simulink model "bh_control_design_sandpit"  (R2016b)
settings: Solver=ode4  StartTime=0.0  StopTime=3  FixedStep=0.001  RelTol=1e-5
libraries: simulink_extras x20, simulink x10, cstblocks x5
settings Model: Creator=bhorton  LastModifiedBy=bhorton
settings SolverCC: ZeroCrossAlgorithm=Adaptive
settings OptimizationCC: LifeSpan=inf
settings DebuggingCC: SFUnexpectedBacktrackingDiag=warning  SFNoUnconditionalDefaultTransitionDiag=warning  SFExecutionAtInitializationDiag=none
settings GRTTargetCC: TargetLangStandard=C89/C90 (ANSI)
settings ConfigComp: CovMetricSettings=dw  CovHtmlReporting=on  CovSaveCumulativeToWorkspaceVar=on  CovSaveSingleToWorkspaceVar=on  CovExternalEMLEnable=off
settings SimscapeCC: SimscapeLogType=all  SimscapeLogDataHistory=10000  SelectedTab=Simscape Multibody
settings ExplorerConfigSet: InternalSimMechanicsExplorerSettings="<ExplorerConfiguration><canonicalview>default</canonicalview><AnimationSetting><BasePlaybackSpeed>1.0</BasePlaybackSpeed><PlaybackSpeedFactor>1.0</PlaybackSpeedFactor></AnimationSetting><TilePanel><TileInfo><Tiles Columns=\"2\" Count=\"4\" Rows=\"2\"><Column Left=\"2\" Weight=\"0.4992\"/><Column Left=\"655\" Weight=\"0.5008\"/><Column Left=\"1310\"/><Row Top=\"2\" Weight=\"0.4984\"/><Row Top=\"475\" Weight=\"0.5016\"/><Row Top=\"950\"/><Tile Height=\"1\" Width=\"1\" X=\"0\" Y=\"0\"/><Tile Height=\"1\" Width=\"1\" X=\"0\" Y=\"1\"/><Tile Height=\"1\" Width=\"1\" X=\"1\" Y=\"0\"/><Tile Height=\"1\" Width=\"1\" X=\"1\" Y=\"1\"/></Tiles></TileInfo><SceneInfo><SceneViewer><BGColor><R>0.60000002384185791</R><G>0.60000002384185791</G><B>0.60000002384185791</B></BGColor><Camera><DoPerspective>off</DoPerspective><Position><X>0.57010570867346566</X><Y>-0.81939487187068383</Y><Z>-0.041325690013103822</Z></Position><Center><X>0.57010570867346566</X><Y>0.37243777720020188</Y><Z>-0.041325690013103822</Z></Center><Up><X>0</X><Y>-0</Y><Z>1</Z></Up><ViewLimDist>1</ViewLimDist><YLim>0.58387397231837834</YLim><XLim>0.8103768064074045</XLim></Camera></SceneViewer><SceneViewer><BGColor><R>0.60000002384185791</R><G>0.60000002384185791</G><B>0.60000002384185791</B></BGColor><Camera><DoPerspective>off</DoPerspective><Position><X>0.51388092361444482</X><Y>0.52196280048326149</Y><Z>0.82022286793681332</Z></Position><Center><X>0.51388092361444482</X><Y>0.52196280048326149</Y><Z>-0.17977713206318668</Z></Center><Up><X>0</X><Y>1</Y><Z>-0</Z></Up><ViewLimDist>1</ViewLimDist><YLim>0.97737746692739225</YLim><XLim>1.3507104907751943</XLim></Camera></SceneViewer><SceneViewer><BGColor><R>0.60000002384185791</R><G>0.60000002384185791</G><B>0.60000002384185791</B></BGColor><Camera><DoPerspective>off</DoPerspective><Position><X>1.5094114010486579</X><Y>0.67796186035410533</Y><Z>-0.0082694811079057073</Z></Position><Center><X>0.47943838776152692</X><Y>0.67796186035410533</Y><Z>-0.0082694811079057073</Z></Center><Up><X>-0</X><Y>0</Y><Z>1</Z></Up><ViewLimDist>1</ViewLimDist><YLim>0.68608550995197048</YLim><XLim>0.95519663670037269</XLim></Camera></SceneViewer><SceneViewer><BGColor><R>0.60000002384185791</R><G>0.60000002384185791</G><B>0.60000002384185791</B></BGColor><Camera><DoPerspective>off</DoPerspective><Position><X>1.2860411296222924</X><Y>0.12259966358168611</Y><Z>0.94383913066063729</Z></Position><Center><X>0.57516484098717713</X><Y>0.83347595221680226</Y><Z>0.23296284202552392</Z></Center><Up><X>-0.40824829046386307</X><Y>0.40824829046386307</Y><Z>0.81649658092772615</Z></Up><ViewLimDist>1</ViewLimDist><YLim>0.94664886749230226</YLim><XLim>1.3123072283262387</XLim></Camera></SceneViewer></SceneInfo></TilePanel><MechEditorPanel><Cameras/><GfxPanelCameraMap/><VideoCreator><PlaybackSpeedRatio>1.0</PlaybackSpeedRatio><FrameRate>30</FrameRate><VideoFormat>Motion JPEG AVI</VideoFormat><FrameSize>auto</FrameSize></VideoCreator></MechEditorPanel></ExplorerConfiguration>"

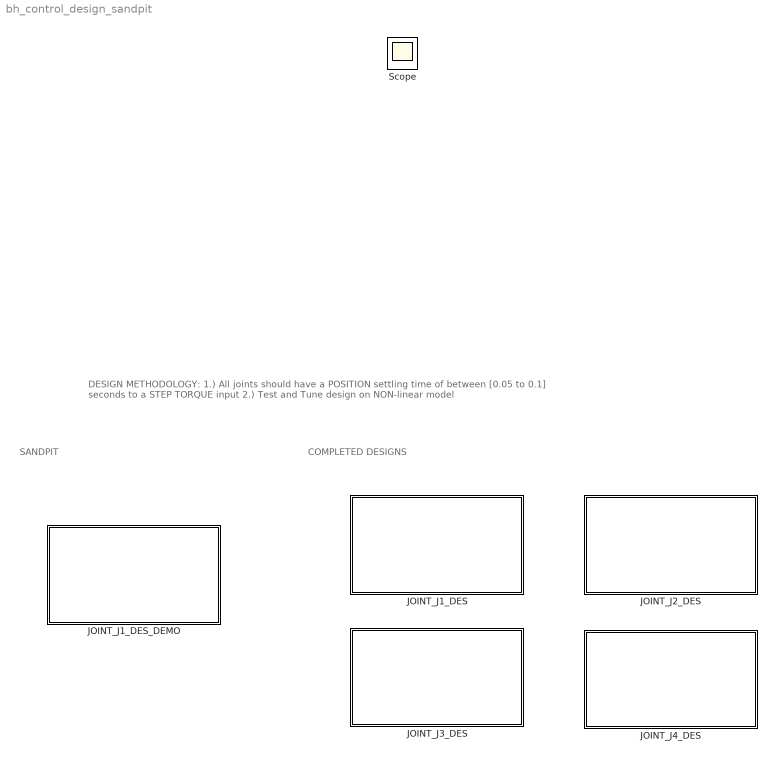
== system bh_control_design_sandpit ==
  note: DESIGN METHODOLOGY:
      | 1.) All joints should have a POSITION settling time of between [0.05 to 0.1] seconds to a STEP TORQUE input
      | 2.) Test and Tune design on NON-linear model
  note: SANDPIT
  note: COMPLETED DESIGNS
  JOINT_J1_DES : Subsystem
  JOINT_J1_DES_DEMO : Subsystem
  JOINT_J2_DES : Subsystem
  JOINT_J3_DES : Subsystem
  JOINT_J4_DES : Subsystem
  Scope : Scope

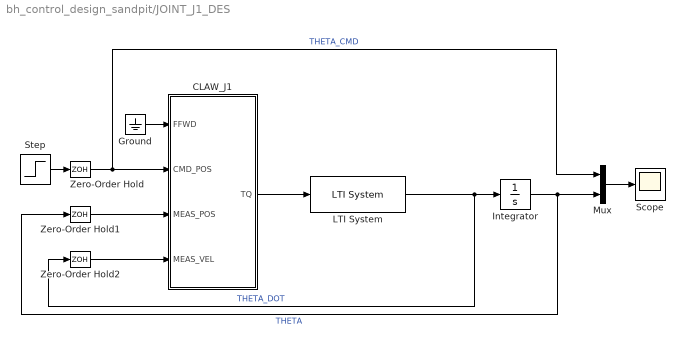
== system bh_control_design_sandpit/JOINT_J1_DES ==
  CLAW_J1 : Subsystem
  Ground : Ground
  Integrator : Integrator
  LTI System : cstblocks/LTI System  sys=TF_J1  IC=[]
  Mux : Mux  Inputs=2
  Scope : Scope
  Step : Step  SampleTime=0
  Zero-Order Hold : ZeroOrderHold  SampleTime=0.001
  Zero-Order Hold1 : ZeroOrderHold  SampleTime=0.001
  Zero-Order Hold2 : ZeroOrderHold  SampleTime=0.001
  wires:
  Ground/1 -> CLAW_J1/1(FFWD)
  Integrator/1 -> Zero-Order Hold1/1, Mux/2  "THETA"
  Mux/1 -> Scope/1
  Step/1 -> Zero-Order Hold/1
  LTI System/1 -> Zero-Order Hold2/1, Integrator/1  "THETA_DOT"
  CLAW_J1/1(TQ) -> LTI System/1
  Zero-Order Hold/1 -> Mux/1, CLAW_J1/2(CMD_POS)  "THETA_CMD"
  Zero-Order Hold1/1 -> CLAW_J1/3(MEAS_POS)
  Zero-Order Hold2/1 -> CLAW_J1/4(MEAS_VEL)

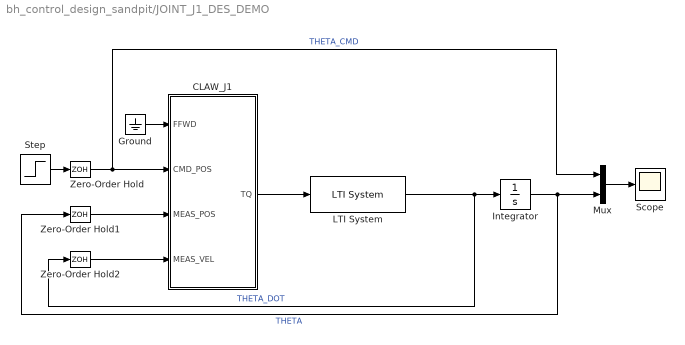
== system bh_control_design_sandpit/JOINT_J1_DES_DEMO ==
  CLAW_J1 : Subsystem
  Ground : Ground
  Integrator : Integrator
  LTI System : cstblocks/LTI System  sys=TF_J1  IC=[]
  Mux : Mux  Inputs=2
  Scope : Scope
  Step : Step  SampleTime=0
  Zero-Order Hold : ZeroOrderHold  SampleTime=0.001
  Zero-Order Hold1 : ZeroOrderHold  SampleTime=0.001
  Zero-Order Hold2 : ZeroOrderHold  SampleTime=0.001
  wires:
  Ground/1 -> CLAW_J1/1(FFWD)
  Integrator/1 -> Zero-Order Hold1/1, Mux/2  "THETA"
  Mux/1 -> Scope/1
  Step/1 -> Zero-Order Hold/1
  LTI System/1 -> Zero-Order Hold2/1, Integrator/1  "THETA_DOT"
  CLAW_J1/1(TQ) -> LTI System/1
  Zero-Order Hold/1 -> Mux/1, CLAW_J1/2(CMD_POS)  "THETA_CMD"
  Zero-Order Hold1/1 -> CLAW_J1/3(MEAS_POS)
  Zero-Order Hold2/1 -> CLAW_J1/4(MEAS_VEL)

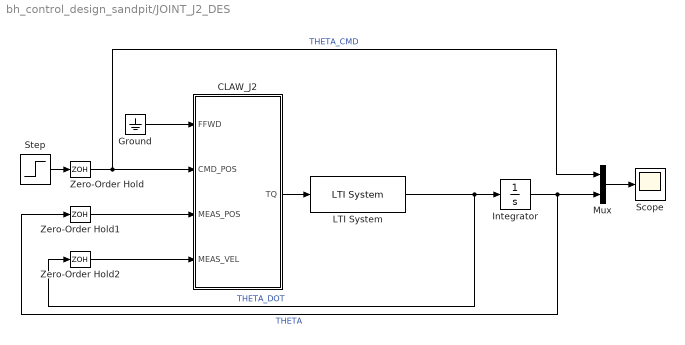
== system bh_control_design_sandpit/JOINT_J2_DES ==
  CLAW_J2 : Subsystem
  Ground : Ground
  Integrator : Integrator
  LTI System : cstblocks/LTI System  sys=TF_J2  IC=[]
  Mux : Mux  Inputs=2
  Scope : Scope
  Step : Step  SampleTime=0
  Zero-Order Hold : ZeroOrderHold  SampleTime=0.001
  Zero-Order Hold1 : ZeroOrderHold  SampleTime=0.001
  Zero-Order Hold2 : ZeroOrderHold  SampleTime=0.001
  wires:
  Ground/1 -> CLAW_J2/1(FFWD)
  Integrator/1 -> Zero-Order Hold1/1, Mux/2  "THETA"
  Mux/1 -> Scope/1
  Step/1 -> Zero-Order Hold/1
  LTI System/1 -> Zero-Order Hold2/1, Integrator/1  "THETA_DOT"
  Zero-Order Hold/1 -> CLAW_J2/2(CMD_POS), Mux/1  "THETA_CMD"
  Zero-Order Hold1/1 -> CLAW_J2/3(MEAS_POS)
  Zero-Order Hold2/1 -> CLAW_J2/4(MEAS_VEL)
  CLAW_J2/1(TQ) -> LTI System/1

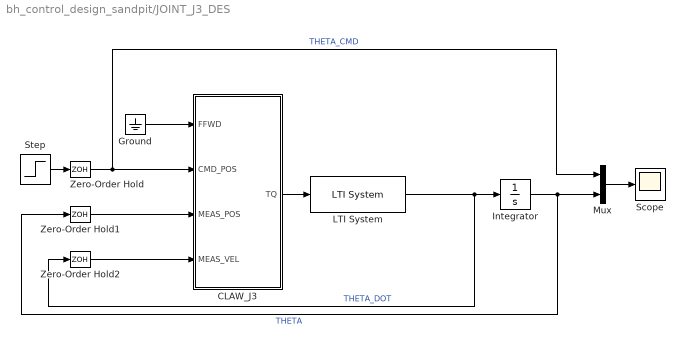
== system bh_control_design_sandpit/JOINT_J3_DES ==
  CLAW_J3 : Subsystem
  Ground : Ground
  Integrator : Integrator
  LTI System : cstblocks/LTI System  sys=TF_J3  IC=[]
  Mux : Mux  Inputs=2
  Scope : Scope
  Step : Step  SampleTime=0
  Zero-Order Hold : ZeroOrderHold  SampleTime=0.001
  Zero-Order Hold1 : ZeroOrderHold  SampleTime=0.001
  Zero-Order Hold2 : ZeroOrderHold  SampleTime=0.001
  wires:
  Ground/1 -> CLAW_J3/1(FFWD)
  Integrator/1 -> Zero-Order Hold1/1, Mux/2  "THETA"
  Mux/1 -> Scope/1
  Step/1 -> Zero-Order Hold/1
  LTI System/1 -> Zero-Order Hold2/1, Integrator/1  "THETA_DOT"
  Zero-Order Hold/1 -> CLAW_J3/2(CMD_POS), Mux/1  "THETA_CMD"
  Zero-Order Hold1/1 -> CLAW_J3/3(MEAS_POS)
  Zero-Order Hold2/1 -> CLAW_J3/4(MEAS_VEL)
  CLAW_J3/1(TQ) -> LTI System/1

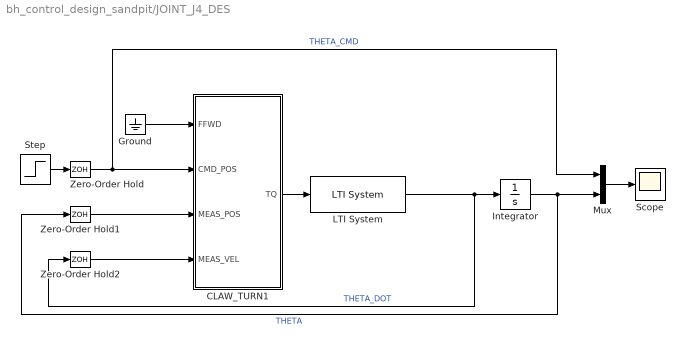
== system bh_control_design_sandpit/JOINT_J4_DES ==
  CLAW_TURN1 : Subsystem
  Ground : Ground
  Integrator : Integrator
  LTI System : cstblocks/LTI System  sys=TF_J4  IC=[]
  Mux : Mux  Inputs=2
  Scope : Scope
  Step : Step  SampleTime=0
  Zero-Order Hold : ZeroOrderHold  SampleTime=0.001
  Zero-Order Hold1 : ZeroOrderHold  SampleTime=0.001
  Zero-Order Hold2 : ZeroOrderHold  SampleTime=0.001
  wires:
  Ground/1 -> CLAW_TURN1/1(FFWD)
  Integrator/1 -> Zero-Order Hold1/1, Mux/2  "THETA"
  Mux/1 -> Scope/1
  Step/1 -> Zero-Order Hold/1
  LTI System/1 -> Zero-Order Hold2/1, Integrator/1  "THETA_DOT"
  Zero-Order Hold/1 -> CLAW_TURN1/2(CMD_POS), Mux/1  "THETA_CMD"
  Zero-Order Hold1/1 -> CLAW_TURN1/3(MEAS_POS)
  Zero-Order Hold2/1 -> CLAW_TURN1/4(MEAS_VEL)
  CLAW_TURN1/1(TQ) -> LTI System/1

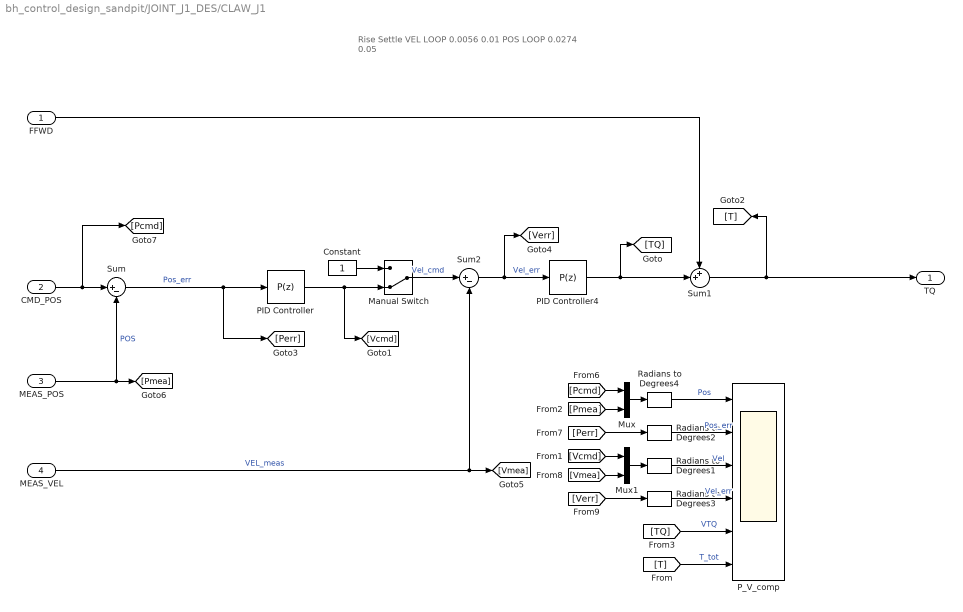
== system bh_control_design_sandpit/JOINT_J1_DES/CLAW_J1 ==
  note: Rise Settle
      | VEL LOOP 0.0056 0.01
      | POS LOOP 0.0274 0.05
  FFWD : Inport
  CMD_POS : Inport  Port=2
  MEAS_POS : Inport  Port=3
  MEAS_VEL : Inport  Port=4
  Constant : Constant
  Manual Switch : ManualSwitch  CurrentSetting=0
  Mux : Mux  Inputs=2
  Mux1 : Mux  Inputs=2
  PID Controller : simulink/Continuous/PID Controller  Controller=P  TimeDomain=Discrete-time  SampleTime=0.001  IntegratorMethod=Forward Euler  FilterMethod=Forward Euler  Form=Parallel  UseFilter=on  ControllerParametersSource=internal  P=69.6165546473111  I=1  D=0  N=100  InitialConditionSource=internal  InitialConditionForIntegrator=0  InitialConditionForFilter=0  ExternalReset=none  LimitOutput=off  UpperSaturationLimit=inf  LowerSaturationLimit=-inf  LinearizeAsGain=on  AntiWindupMode=none  Kb=1  TrackingMode=off  Kt=1  PParamMin=[]  PParamMax=[]  IParamMin=[]  IParamMax=[]  DParamMin=[]  DParamMax=[]  NParamMin=[]  NParamMax=[]  KbParamMin=[]  KbParamMax=[]  KtParamMin=[]  KtParamMax=[]  POutMin=[]  POutMax=[]  IOutMin=[]  IOutMax=[]  DOutMin=[]  DOutMax=[]  NOutMin=[]  NOutMax=[]  KbOutMin=[]  KbOutMax=[]  KtOutMin=[]  KtOutMax=[]  IntegratorOutMin=[]  IntegratorOutMax=[]  FilterOutMin=[]  FilterOutMax=[]  SumOutMin=[]  SumOutMax=[]  SumI1OutMin=[]  SumI1OutMax=[]  SumI2OutMin=[]  SumI2OutMax=[]  SumI3OutMin=[]  SumI3OutMax=[]  SumDOutMin=[]  SumDOutMax=[]  SaturationOutMin=[]  SaturationOutMax=[]  IntegratorContinuousStateAttributes=''  IntegratorStateMustResolveToSignalObject=off  IntegratorRTWStateStorageClass=Auto  FilterContinuousStateAttributes=''  FilterStateMustResolveToSignalObject=off  FilterRTWStateStorageClass=Auto  DifferentiatorICPrevScaledInput=0  DifferentiatorOutMin=[]  DifferentiatorOutMax=[]
      settings: AttributesFormatString=DT= %<SampleTime>
  PID Controller4 : simulink/Continuous/PID Controller  Controller=P  TimeDomain=Discrete-time  SampleTime=0.001  IntegratorMethod=Forward Euler  FilterMethod=Forward Euler  Form=Parallel  UseFilter=on  ControllerParametersSource=internal  P=33.613608015401  I=10  D=0  N=100  InitialConditionSource=internal  InitialConditionForIntegrator=0  InitialConditionForFilter=0  ExternalReset=none  LimitOutput=off  UpperSaturationLimit=inf  LowerSaturationLimit=-inf  LinearizeAsGain=on  AntiWindupMode=none  Kb=1  TrackingMode=off  Kt=1  PParamMin=[]  PParamMax=[]  IParamMin=[]  IParamMax=[]  DParamMin=[]  DParamMax=[]  NParamMin=[]  NParamMax=[]  KbParamMin=[]  KbParamMax=[]  KtParamMin=[]  KtParamMax=[]  POutMin=[]  POutMax=[]  IOutMin=[]  IOutMax=[]  DOutMin=[]  DOutMax=[]  NOutMin=[]  NOutMax=[]  KbOutMin=[]  KbOutMax=[]  KtOutMin=[]  KtOutMax=[]  IntegratorOutMin=[]  IntegratorOutMax=[]  FilterOutMin=[]  FilterOutMax=[]  SumOutMin=[]  SumOutMax=[]  SumI1OutMin=[]  SumI1OutMax=[]  SumI2OutMin=[]  SumI2OutMax=[]  SumI3OutMin=[]  SumI3OutMax=[]  SumDOutMin=[]  SumDOutMax=[]  SaturationOutMin=[]  SaturationOutMax=[]  IntegratorContinuousStateAttributes=''  IntegratorStateMustResolveToSignalObject=off  IntegratorRTWStateStorageClass=Auto  FilterContinuousStateAttributes=''  FilterStateMustResolveToSignalObject=off  FilterRTWStateStorageClass=Auto  DifferentiatorICPrevScaledInput=0  DifferentiatorOutMin=[]  DifferentiatorOutMax=[]
      settings: AttributesFormatString=DT= %<SampleTime>
  P_V_comp : Scope  NumInputPorts=6
  Radians to Degrees{1..4} (4 alike) : simulink_extras/Transformations/Radians to Degrees
  Sum : Sum  Inputs=|+-
  Sum1 : Sum  Inputs=++|
  Sum2 : Sum  Inputs=|+-
  TQ : Outport
  wires:
  FFWD/1 -> Sum1/1
  CMD_POS/1 -> [Pcmd], Sum/1
  MEAS_POS/1 -> [Pmea], Sum/2  "POS"
  Sum2/1 -> PID Controller4/1, [Verr]  "Vel_err"
  Manual Switch/1 -> Sum2/1  "Vel_cmd"
  Constant/1 -> Manual Switch/1
  Sum/1 -> PID Controller/1, [Perr]  "Pos_err"
  PID Controller/1 -> Manual Switch/2, [Vcmd]
  Sum1/1 -> TQ/1, [T]
  Mux/1 -> Radians to Degrees4/1
  [Pcmd] -> Mux/1
  [Pmea] -> Mux/2
  Mux1/1 -> Radians to Degrees1/1
  [Vcmd] -> Mux1/1
  [Vmea] -> Mux1/2
  [Verr] -> Radians to Degrees3/1
  [Perr] -> Radians to Degrees2/1
  Radians to Degrees3/1 -> P_V_comp/4  "Vel_err"
  Radians to Degrees2/1 -> P_V_comp/2  "Pos_err"
  Radians to Degrees1/1 -> P_V_comp/3  "Vel"
  Radians to Degrees4/1 -> P_V_comp/1  "Pos"
  [TQ] -> P_V_comp/5  "VTQ"
  [T] -> P_V_comp/6  "T_tot"
  PID Controller4/1 -> Sum1/2, [TQ]
  MEAS_VEL/1 -> Sum2/2, [Vmea]  "VEL_meas"

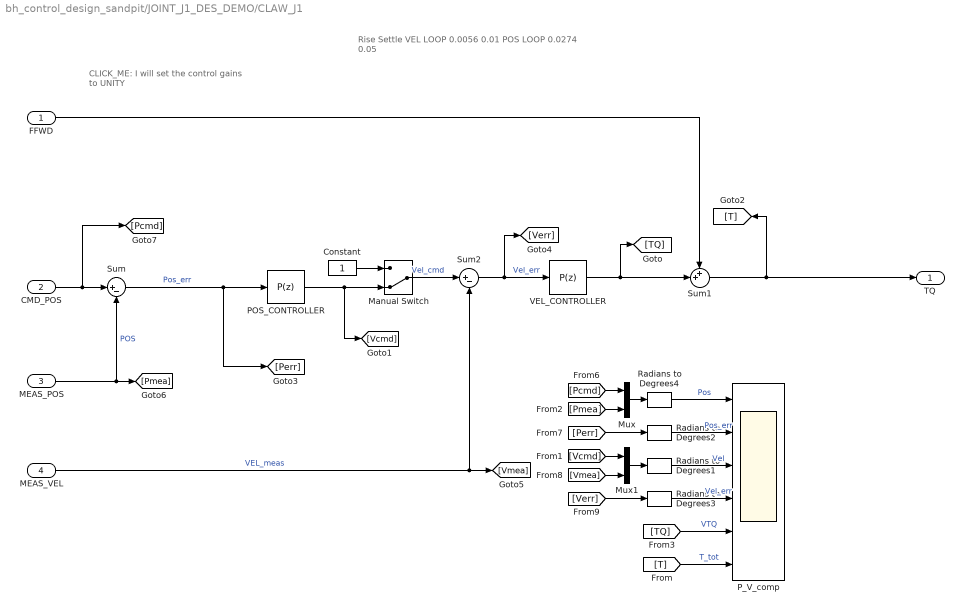
== system bh_control_design_sandpit/JOINT_J1_DES_DEMO/CLAW_J1 ==
  note: CLICK_ME:
      | I will set the control gains to UNITY
  note: Rise Settle
      | VEL LOOP 0.0056 0.01
      | POS LOOP 0.0274 0.05
  FFWD : Inport
  CMD_POS : Inport  Port=2
  MEAS_POS : Inport  Port=3
  MEAS_VEL : Inport  Port=4
  Constant : Constant
  Manual Switch : ManualSwitch  CurrentSetting=0
  Mux : Mux  Inputs=2
  Mux1 : Mux  Inputs=2
  POS_CONTROLLER : simulink/Continuous/PID Controller  Controller=P  TimeDomain=Discrete-time  SampleTime=0.001  IntegratorMethod=Forward Euler  FilterMethod=Forward Euler  Form=Parallel  UseFilter=on  ControllerParametersSource=internal  P=1  I=1  D=0  N=100  InitialConditionSource=internal  InitialConditionForIntegrator=0  InitialConditionForFilter=0  ExternalReset=none  LimitOutput=off  UpperSaturationLimit=inf  LowerSaturationLimit=-inf  LinearizeAsGain=on  AntiWindupMode=none  Kb=1  TrackingMode=off  Kt=1  PParamMin=[]  PParamMax=[]  IParamMin=[]  IParamMax=[]  DParamMin=[]  DParamMax=[]  NParamMin=[]  NParamMax=[]  KbParamMin=[]  KbParamMax=[]  KtParamMin=[]  KtParamMax=[]  POutMin=[]  POutMax=[]  IOutMin=[]  IOutMax=[]  DOutMin=[]  DOutMax=[]  NOutMin=[]  NOutMax=[]  KbOutMin=[]  KbOutMax=[]  KtOutMin=[]  KtOutMax=[]  IntegratorOutMin=[]  IntegratorOutMax=[]  FilterOutMin=[]  FilterOutMax=[]  SumOutMin=[]  SumOutMax=[]  SumI1OutMin=[]  SumI1OutMax=[]  SumI2OutMin=[]  SumI2OutMax=[]  SumI3OutMin=[]  SumI3OutMax=[]  SumDOutMin=[]  SumDOutMax=[]  SaturationOutMin=[]  SaturationOutMax=[]  IntegratorContinuousStateAttributes=''  IntegratorStateMustResolveToSignalObject=off  IntegratorRTWStateStorageClass=Auto  FilterContinuousStateAttributes=''  FilterStateMustResolveToSignalObject=off  FilterRTWStateStorageClass=Auto  DifferentiatorICPrevScaledInput=0  DifferentiatorOutMin=[]  DifferentiatorOutMax=[]
      settings: AttributesFormatString=|
      | DT= %<SampleTime>
      | P = %<P>
  P_V_comp : Scope  NumInputPorts=6
  Radians to Degrees{1..4} (4 alike) : simulink_extras/Transformations/Radians to Degrees
  Sum : Sum  Inputs=|+-
  Sum1 : Sum  Inputs=++|
  Sum2 : Sum  Inputs=|+-
  VEL_CONTROLLER : simulink/Continuous/PID Controller  Controller=P  TimeDomain=Discrete-time  SampleTime=0.001  IntegratorMethod=Forward Euler  FilterMethod=Forward Euler  Form=Parallel  UseFilter=on  ControllerParametersSource=internal  P=1  I=10  D=0  N=100  InitialConditionSource=internal  InitialConditionForIntegrator=0  InitialConditionForFilter=0  ExternalReset=none  LimitOutput=off  UpperSaturationLimit=inf  LowerSaturationLimit=-inf  LinearizeAsGain=on  AntiWindupMode=none  Kb=1  TrackingMode=off  Kt=1  PParamMin=[]  PParamMax=[]  IParamMin=[]  IParamMax=[]  DParamMin=[]  DParamMax=[]  NParamMin=[]  NParamMax=[]  KbParamMin=[]  KbParamMax=[]  KtParamMin=[]  KtParamMax=[]  POutMin=[]  POutMax=[]  IOutMin=[]  IOutMax=[]  DOutMin=[]  DOutMax=[]  NOutMin=[]  NOutMax=[]  KbOutMin=[]  KbOutMax=[]  KtOutMin=[]  KtOutMax=[]  IntegratorOutMin=[]  IntegratorOutMax=[]  FilterOutMin=[]  FilterOutMax=[]  SumOutMin=[]  SumOutMax=[]  SumI1OutMin=[]  SumI1OutMax=[]  SumI2OutMin=[]  SumI2OutMax=[]  SumI3OutMin=[]  SumI3OutMax=[]  SumDOutMin=[]  SumDOutMax=[]  SaturationOutMin=[]  SaturationOutMax=[]  IntegratorContinuousStateAttributes=''  IntegratorStateMustResolveToSignalObject=off  IntegratorRTWStateStorageClass=Auto  FilterContinuousStateAttributes=''  FilterStateMustResolveToSignalObject=off  FilterRTWStateStorageClass=Auto  DifferentiatorICPrevScaledInput=0  DifferentiatorOutMin=[]  DifferentiatorOutMax=[]
      settings: AttributesFormatString=|
      | DT= %<SampleTime>
      | P = %<P>
  TQ : Outport
  wires:
  FFWD/1 -> Sum1/1
  CMD_POS/1 -> [Pcmd], Sum/1
  MEAS_POS/1 -> [Pmea], Sum/2  "POS"
  Sum2/1 -> VEL_CONTROLLER/1, [Verr]  "Vel_err"
  Manual Switch/1 -> Sum2/1  "Vel_cmd"
  Constant/1 -> Manual Switch/1
  Sum/1 -> POS_CONTROLLER/1, [Perr]  "Pos_err"
  POS_CONTROLLER/1 -> Manual Switch/2, [Vcmd]
  Sum1/1 -> TQ/1, [T]
  Mux/1 -> Radians to Degrees4/1
  [Pcmd] -> Mux/1
  [Pmea] -> Mux/2
  Mux1/1 -> Radians to Degrees1/1
  [Vcmd] -> Mux1/1
  [Vmea] -> Mux1/2
  [Verr] -> Radians to Degrees3/1
  [Perr] -> Radians to Degrees2/1
  Radians to Degrees3/1 -> P_V_comp/4  "Vel_err"
  Radians to Degrees2/1 -> P_V_comp/2  "Pos_err"
  Radians to Degrees1/1 -> P_V_comp/3  "Vel"
  Radians to Degrees4/1 -> P_V_comp/1  "Pos"
  [TQ] -> P_V_comp/5  "VTQ"
  [T] -> P_V_comp/6  "T_tot"
  VEL_CONTROLLER/1 -> Sum1/2, [TQ]
  MEAS_VEL/1 -> Sum2/2, [Vmea]  "VEL_meas"

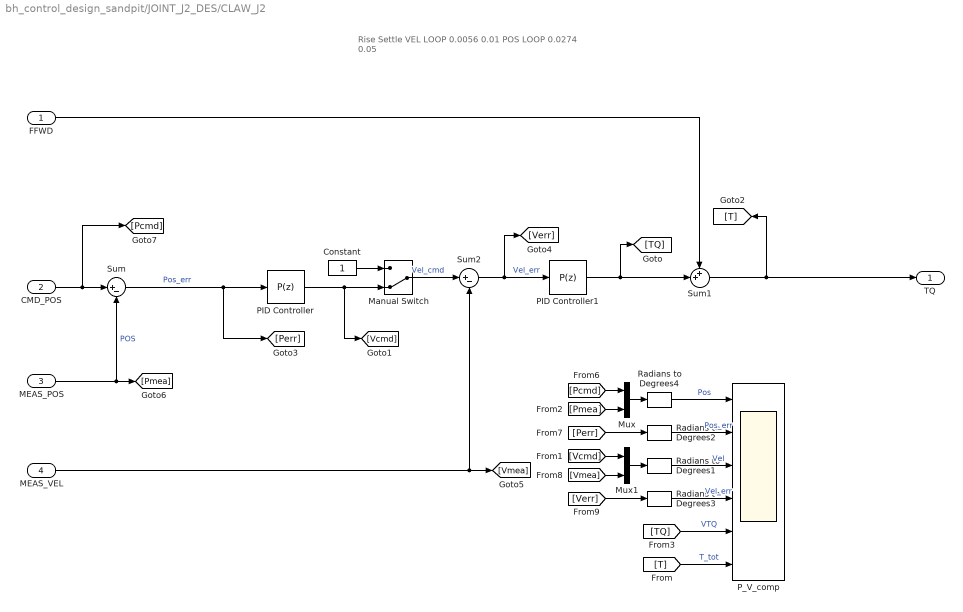
== system bh_control_design_sandpit/JOINT_J2_DES/CLAW_J2 ==
  note: Rise Settle
      | VEL LOOP 0.0056 0.01
      | POS LOOP 0.0274 0.05
  FFWD : Inport
  CMD_POS : Inport  Port=2
  MEAS_POS : Inport  Port=3
  MEAS_VEL : Inport  Port=4
  Constant : Constant
  Manual Switch : ManualSwitch  CurrentSetting=0
  Mux : Mux  Inputs=2
  Mux1 : Mux  Inputs=2
  PID Controller : simulink/Continuous/PID Controller  Controller=P  TimeDomain=Discrete-time  SampleTime=0.001  IntegratorMethod=Forward Euler  FilterMethod=Forward Euler  Form=Parallel  UseFilter=on  ControllerParametersSource=internal  P=73.0033216237391  I=1  D=0  N=100  InitialConditionSource=internal  InitialConditionForIntegrator=0  InitialConditionForFilter=0  ExternalReset=none  LimitOutput=off  UpperSaturationLimit=inf  LowerSaturationLimit=-inf  LinearizeAsGain=on  AntiWindupMode=none  Kb=1  TrackingMode=off  Kt=1  PParamMin=[]  PParamMax=[]  IParamMin=[]  IParamMax=[]  DParamMin=[]  DParamMax=[]  NParamMin=[]  NParamMax=[]  KbParamMin=[]  KbParamMax=[]  KtParamMin=[]  KtParamMax=[]  POutMin=[]  POutMax=[]  IOutMin=[]  IOutMax=[]  DOutMin=[]  DOutMax=[]  NOutMin=[]  NOutMax=[]  KbOutMin=[]  KbOutMax=[]  KtOutMin=[]  KtOutMax=[]  IntegratorOutMin=[]  IntegratorOutMax=[]  FilterOutMin=[]  FilterOutMax=[]  SumOutMin=[]  SumOutMax=[]  SumI1OutMin=[]  SumI1OutMax=[]  SumI2OutMin=[]  SumI2OutMax=[]  SumI3OutMin=[]  SumI3OutMax=[]  SumDOutMin=[]  SumDOutMax=[]  SaturationOutMin=[]  SaturationOutMax=[]  IntegratorContinuousStateAttributes=''  IntegratorStateMustResolveToSignalObject=off  IntegratorRTWStateStorageClass=Auto  FilterContinuousStateAttributes=''  FilterStateMustResolveToSignalObject=off  FilterRTWStateStorageClass=Auto  DifferentiatorICPrevScaledInput=0  DifferentiatorOutMin=[]  DifferentiatorOutMax=[]
      settings: AttributesFormatString=DT= %<SampleTime>
  PID Controller1 : simulink/Continuous/PID Controller  Controller=P  TimeDomain=Discrete-time  SampleTime=0.001  IntegratorMethod=Forward Euler  FilterMethod=Forward Euler  Form=Parallel  UseFilter=on  ControllerParametersSource=internal  P=3.67375636906799  I=10  D=0  N=100  InitialConditionSource=internal  InitialConditionForIntegrator=0  InitialConditionForFilter=0  ExternalReset=none  LimitOutput=off  UpperSaturationLimit=inf  LowerSaturationLimit=-inf  LinearizeAsGain=on  AntiWindupMode=none  Kb=1  TrackingMode=off  Kt=1  PParamMin=[]  PParamMax=[]  IParamMin=[]  IParamMax=[]  DParamMin=[]  DParamMax=[]  NParamMin=[]  NParamMax=[]  KbParamMin=[]  KbParamMax=[]  KtParamMin=[]  KtParamMax=[]  POutMin=[]  POutMax=[]  IOutMin=[]  IOutMax=[]  DOutMin=[]  DOutMax=[]  NOutMin=[]  NOutMax=[]  KbOutMin=[]  KbOutMax=[]  KtOutMin=[]  KtOutMax=[]  IntegratorOutMin=[]  IntegratorOutMax=[]  FilterOutMin=[]  FilterOutMax=[]  SumOutMin=[]  SumOutMax=[]  SumI1OutMin=[]  SumI1OutMax=[]  SumI2OutMin=[]  SumI2OutMax=[]  SumI3OutMin=[]  SumI3OutMax=[]  SumDOutMin=[]  SumDOutMax=[]  SaturationOutMin=[]  SaturationOutMax=[]  IntegratorContinuousStateAttributes=''  IntegratorStateMustResolveToSignalObject=off  IntegratorRTWStateStorageClass=Auto  FilterContinuousStateAttributes=''  FilterStateMustResolveToSignalObject=off  FilterRTWStateStorageClass=Auto  DifferentiatorICPrevScaledInput=0  DifferentiatorOutMin=[]  DifferentiatorOutMax=[]
      settings: AttributesFormatString=DT= %<SampleTime>
  P_V_comp : Scope  NumInputPorts=6
  Radians to Degrees{1..4} (4 alike) : simulink_extras/Transformations/Radians to Degrees
  Sum : Sum  Inputs=|+-
  Sum1 : Sum  Inputs=++|
  Sum2 : Sum  Inputs=|+-
  TQ : Outport
  wires:
  FFWD/1 -> Sum1/1
  CMD_POS/1 -> [Pcmd], Sum/1
  MEAS_POS/1 -> [Pmea], Sum/2  "POS"
  Sum2/1 -> PID Controller1/1, [Verr]  "Vel_err"
  Manual Switch/1 -> Sum2/1  "Vel_cmd"
  Constant/1 -> Manual Switch/1
  Sum/1 -> PID Controller/1, [Perr]  "Pos_err"
  PID Controller/1 -> Manual Switch/2, [Vcmd]
  Sum1/1 -> TQ/1, [T]
  Mux/1 -> Radians to Degrees4/1
  [Pcmd] -> Mux/1
  [Pmea] -> Mux/2
  Mux1/1 -> Radians to Degrees1/1
  [Vcmd] -> Mux1/1
  [Vmea] -> Mux1/2
  [Verr] -> Radians to Degrees3/1
  [Perr] -> Radians to Degrees2/1
  Radians to Degrees3/1 -> P_V_comp/4  "Vel_err"
  Radians to Degrees2/1 -> P_V_comp/2  "Pos_err"
  Radians to Degrees1/1 -> P_V_comp/3  "Vel"
  Radians to Degrees4/1 -> P_V_comp/1  "Pos"
  [TQ] -> P_V_comp/5  "VTQ"
  [T] -> P_V_comp/6  "T_tot"
  PID Controller1/1 -> Sum1/2, [TQ]
  MEAS_VEL/1 -> [Vmea], Sum2/2

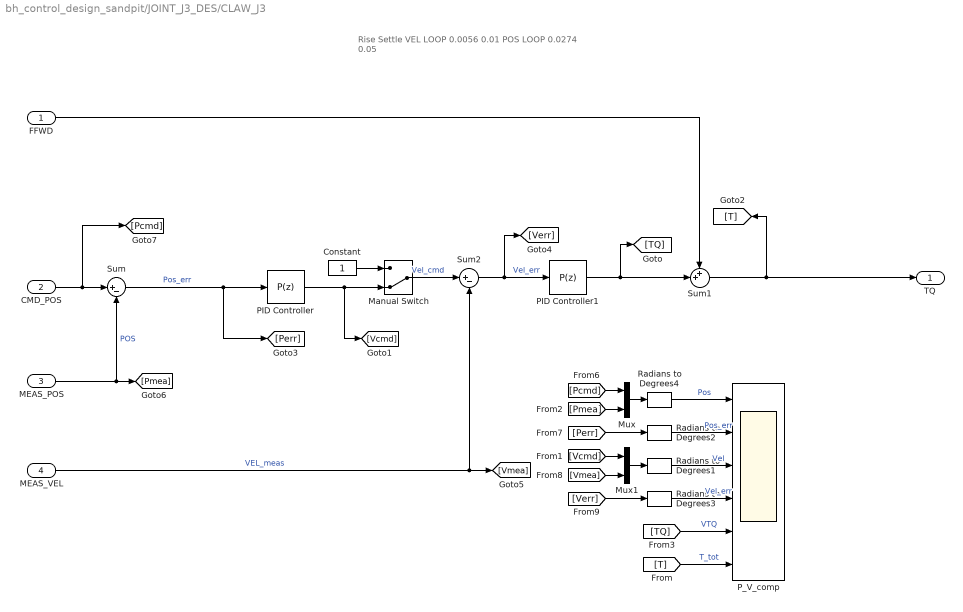
== system bh_control_design_sandpit/JOINT_J3_DES/CLAW_J3 ==
  note: Rise Settle
      | VEL LOOP 0.0056 0.01
      | POS LOOP 0.0274 0.05
  FFWD : Inport
  CMD_POS : Inport  Port=2
  MEAS_POS : Inport  Port=3
  MEAS_VEL : Inport  Port=4
  Constant : Constant
  Manual Switch : ManualSwitch  CurrentSetting=0
  Mux : Mux  Inputs=2
  Mux1 : Mux  Inputs=2
  PID Controller : simulink/Continuous/PID Controller  Controller=P  TimeDomain=Discrete-time  SampleTime=0.001  IntegratorMethod=Forward Euler  FilterMethod=Forward Euler  Form=Parallel  UseFilter=on  ControllerParametersSource=internal  P=76.8539388494415  I=1  D=0  N=100  InitialConditionSource=internal  InitialConditionForIntegrator=0  InitialConditionForFilter=0  ExternalReset=none  LimitOutput=off  UpperSaturationLimit=inf  LowerSaturationLimit=-inf  LinearizeAsGain=on  AntiWindupMode=none  Kb=1  TrackingMode=off  Kt=1  PParamMin=[]  PParamMax=[]  IParamMin=[]  IParamMax=[]  DParamMin=[]  DParamMax=[]  NParamMin=[]  NParamMax=[]  KbParamMin=[]  KbParamMax=[]  KtParamMin=[]  KtParamMax=[]  POutMin=[]  POutMax=[]  IOutMin=[]  IOutMax=[]  DOutMin=[]  DOutMax=[]  NOutMin=[]  NOutMax=[]  KbOutMin=[]  KbOutMax=[]  KtOutMin=[]  KtOutMax=[]  IntegratorOutMin=[]  IntegratorOutMax=[]  FilterOutMin=[]  FilterOutMax=[]  SumOutMin=[]  SumOutMax=[]  SumI1OutMin=[]  SumI1OutMax=[]  SumI2OutMin=[]  SumI2OutMax=[]  SumI3OutMin=[]  SumI3OutMax=[]  SumDOutMin=[]  SumDOutMax=[]  SaturationOutMin=[]  SaturationOutMax=[]  IntegratorContinuousStateAttributes=''  IntegratorStateMustResolveToSignalObject=off  IntegratorRTWStateStorageClass=Auto  FilterContinuousStateAttributes=''  FilterStateMustResolveToSignalObject=off  FilterRTWStateStorageClass=Auto  DifferentiatorICPrevScaledInput=0  DifferentiatorOutMin=[]  DifferentiatorOutMax=[]
      settings: AttributesFormatString=DT= %<SampleTime>
  PID Controller1 : simulink/Continuous/PID Controller  Controller=P  TimeDomain=Discrete-time  SampleTime=0.001  IntegratorMethod=Forward Euler  FilterMethod=Forward Euler  Form=Parallel  UseFilter=on  ControllerParametersSource=internal  P=0.428197184967293  I=10  D=0  N=100  InitialConditionSource=internal  InitialConditionForIntegrator=0  InitialConditionForFilter=0  ExternalReset=none  LimitOutput=off  UpperSaturationLimit=inf  LowerSaturationLimit=-inf  LinearizeAsGain=on  AntiWindupMode=none  Kb=1  TrackingMode=off  Kt=1  PParamMin=[]  PParamMax=[]  IParamMin=[]  IParamMax=[]  DParamMin=[]  DParamMax=[]  NParamMin=[]  NParamMax=[]  KbParamMin=[]  KbParamMax=[]  KtParamMin=[]  KtParamMax=[]  POutMin=[]  POutMax=[]  IOutMin=[]  IOutMax=[]  DOutMin=[]  DOutMax=[]  NOutMin=[]  NOutMax=[]  KbOutMin=[]  KbOutMax=[]  KtOutMin=[]  KtOutMax=[]  IntegratorOutMin=[]  IntegratorOutMax=[]  FilterOutMin=[]  FilterOutMax=[]  SumOutMin=[]  SumOutMax=[]  SumI1OutMin=[]  SumI1OutMax=[]  SumI2OutMin=[]  SumI2OutMax=[]  SumI3OutMin=[]  SumI3OutMax=[]  SumDOutMin=[]  SumDOutMax=[]  SaturationOutMin=[]  SaturationOutMax=[]  IntegratorContinuousStateAttributes=''  IntegratorStateMustResolveToSignalObject=off  IntegratorRTWStateStorageClass=Auto  FilterContinuousStateAttributes=''  FilterStateMustResolveToSignalObject=off  FilterRTWStateStorageClass=Auto  DifferentiatorICPrevScaledInput=0  DifferentiatorOutMin=[]  DifferentiatorOutMax=[]
      settings: AttributesFormatString=DT= %<SampleTime>
  P_V_comp : Scope  NumInputPorts=6
  Radians to Degrees{1..4} (4 alike) : simulink_extras/Transformations/Radians to Degrees
  Sum : Sum  Inputs=|+-
  Sum1 : Sum  Inputs=++|
  Sum2 : Sum  Inputs=|+-
  TQ : Outport
  wires:
  FFWD/1 -> Sum1/1
  CMD_POS/1 -> [Pcmd], Sum/1
  MEAS_VEL/1 -> [Vmea], Sum2/2  "VEL_meas"
  MEAS_POS/1 -> [Pmea], Sum/2  "POS"
  Sum2/1 -> PID Controller1/1, [Verr]  "Vel_err"
  Manual Switch/1 -> Sum2/1  "Vel_cmd"
  Constant/1 -> Manual Switch/1
  Sum/1 -> PID Controller/1, [Perr]  "Pos_err"
  PID Controller/1 -> Manual Switch/2, [Vcmd]
  Sum1/1 -> TQ/1, [T]
  Mux/1 -> Radians to Degrees4/1
  [Pcmd] -> Mux/1
  [Pmea] -> Mux/2
  Mux1/1 -> Radians to Degrees1/1
  [Vcmd] -> Mux1/1
  [Vmea] -> Mux1/2
  [Verr] -> Radians to Degrees3/1
  [Perr] -> Radians to Degrees2/1
  Radians to Degrees3/1 -> P_V_comp/4  "Vel_err"
  Radians to Degrees2/1 -> P_V_comp/2  "Pos_err"
  Radians to Degrees1/1 -> P_V_comp/3  "Vel"
  Radians to Degrees4/1 -> P_V_comp/1  "Pos"
  [TQ] -> P_V_comp/5  "VTQ"
  [T] -> P_V_comp/6  "T_tot"
  PID Controller1/1 -> Sum1/2, [TQ]

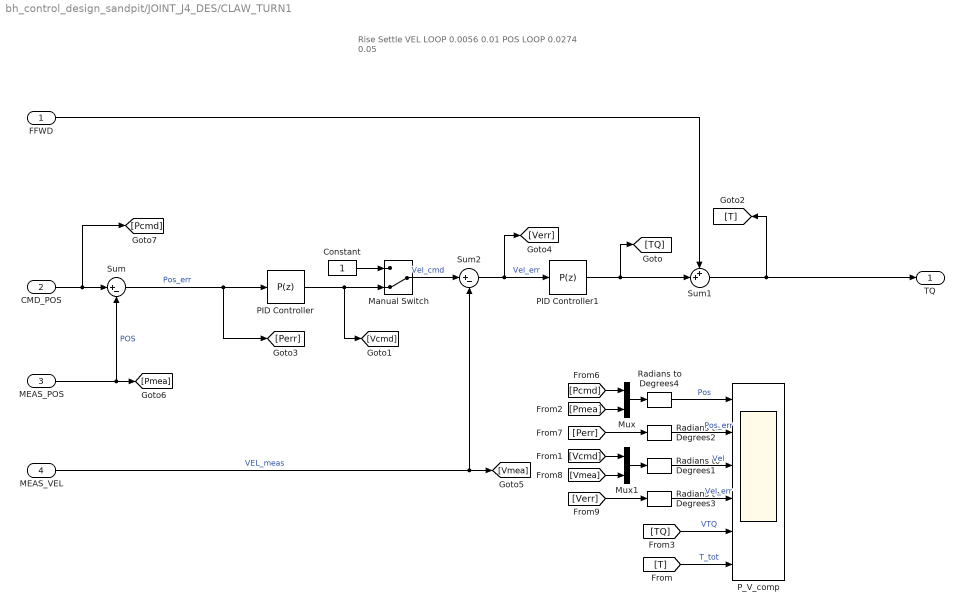
== system bh_control_design_sandpit/JOINT_J4_DES/CLAW_TURN1 ==
  note: Rise Settle
      | VEL LOOP 0.0056 0.01
      | POS LOOP 0.0274 0.05
  FFWD : Inport
  CMD_POS : Inport  Port=2
  MEAS_POS : Inport  Port=3
  MEAS_VEL : Inport  Port=4
  Constant : Constant
  Manual Switch : ManualSwitch  CurrentSetting=0
  Mux : Mux  Inputs=2
  Mux1 : Mux  Inputs=2
  PID Controller : simulink/Continuous/PID Controller  Controller=P  TimeDomain=Discrete-time  SampleTime=0.001  IntegratorMethod=Forward Euler  FilterMethod=Forward Euler  Form=Parallel  UseFilter=on  ControllerParametersSource=internal  P=63.4743382439453  I=1  D=0  N=100  InitialConditionSource=internal  InitialConditionForIntegrator=0  InitialConditionForFilter=0  ExternalReset=none  LimitOutput=off  UpperSaturationLimit=inf  LowerSaturationLimit=-inf  LinearizeAsGain=on  AntiWindupMode=none  Kb=1  TrackingMode=off  Kt=1  PParamMin=[]  PParamMax=[]  IParamMin=[]  IParamMax=[]  DParamMin=[]  DParamMax=[]  NParamMin=[]  NParamMax=[]  KbParamMin=[]  KbParamMax=[]  KtParamMin=[]  KtParamMax=[]  POutMin=[]  POutMax=[]  IOutMin=[]  IOutMax=[]  DOutMin=[]  DOutMax=[]  NOutMin=[]  NOutMax=[]  KbOutMin=[]  KbOutMax=[]  KtOutMin=[]  KtOutMax=[]  IntegratorOutMin=[]  IntegratorOutMax=[]  FilterOutMin=[]  FilterOutMax=[]  SumOutMin=[]  SumOutMax=[]  SumI1OutMin=[]  SumI1OutMax=[]  SumI2OutMin=[]  SumI2OutMax=[]  SumI3OutMin=[]  SumI3OutMax=[]  SumDOutMin=[]  SumDOutMax=[]  SaturationOutMin=[]  SaturationOutMax=[]  IntegratorContinuousStateAttributes=''  IntegratorStateMustResolveToSignalObject=off  IntegratorRTWStateStorageClass=Auto  FilterContinuousStateAttributes=''  FilterStateMustResolveToSignalObject=off  FilterRTWStateStorageClass=Auto  DifferentiatorICPrevScaledInput=0  DifferentiatorOutMin=[]  DifferentiatorOutMax=[]
      settings: AttributesFormatString=DT= %<SampleTime>
  PID Controller1 : simulink/Continuous/PID Controller  Controller=P  TimeDomain=Discrete-time  SampleTime=0.001  IntegratorMethod=Forward Euler  FilterMethod=Forward Euler  Form=Parallel  UseFilter=on  ControllerParametersSource=internal  P=92.748831049679  I=10  D=0  N=100  InitialConditionSource=internal  InitialConditionForIntegrator=0  InitialConditionForFilter=0  ExternalReset=none  LimitOutput=off  UpperSaturationLimit=inf  LowerSaturationLimit=-inf  LinearizeAsGain=on  AntiWindupMode=none  Kb=1  TrackingMode=off  Kt=1  PParamMin=[]  PParamMax=[]  IParamMin=[]  IParamMax=[]  DParamMin=[]  DParamMax=[]  NParamMin=[]  NParamMax=[]  KbParamMin=[]  KbParamMax=[]  KtParamMin=[]  KtParamMax=[]  POutMin=[]  POutMax=[]  IOutMin=[]  IOutMax=[]  DOutMin=[]  DOutMax=[]  NOutMin=[]  NOutMax=[]  KbOutMin=[]  KbOutMax=[]  KtOutMin=[]  KtOutMax=[]  IntegratorOutMin=[]  IntegratorOutMax=[]  FilterOutMin=[]  FilterOutMax=[]  SumOutMin=[]  SumOutMax=[]  SumI1OutMin=[]  SumI1OutMax=[]  SumI2OutMin=[]  SumI2OutMax=[]  SumI3OutMin=[]  SumI3OutMax=[]  SumDOutMin=[]  SumDOutMax=[]  SaturationOutMin=[]  SaturationOutMax=[]  IntegratorContinuousStateAttributes=''  IntegratorStateMustResolveToSignalObject=off  IntegratorRTWStateStorageClass=Auto  FilterContinuousStateAttributes=''  FilterStateMustResolveToSignalObject=off  FilterRTWStateStorageClass=Auto  DifferentiatorICPrevScaledInput=0  DifferentiatorOutMin=[]  DifferentiatorOutMax=[]
      settings: AttributesFormatString=DT= %<SampleTime>
  P_V_comp : Scope  NumInputPorts=6
  Radians to Degrees{1..4} (4 alike) : simulink_extras/Transformations/Radians to Degrees
  Sum : Sum  Inputs=|+-
  Sum1 : Sum  Inputs=++|
  Sum2 : Sum  Inputs=|+-
  TQ : Outport
  wires:
  FFWD/1 -> Sum1/1
  CMD_POS/1 -> [Pcmd], Sum/1
  MEAS_VEL/1 -> [Vmea], Sum2/2  "VEL_meas"
  MEAS_POS/1 -> [Pmea], Sum/2  "POS"
  Sum2/1 -> PID Controller1/1, [Verr]  "Vel_err"
  Manual Switch/1 -> Sum2/1  "Vel_cmd"
  Constant/1 -> Manual Switch/1
  Sum/1 -> PID Controller/1, [Perr]  "Pos_err"
  PID Controller/1 -> Manual Switch/2, [Vcmd]
  Sum1/1 -> TQ/1, [T]
  Mux/1 -> Radians to Degrees4/1
  [Pcmd] -> Mux/1
  [Pmea] -> Mux/2
  Mux1/1 -> Radians to Degrees1/1
  [Vcmd] -> Mux1/1
  [Vmea] -> Mux1/2
  [Verr] -> Radians to Degrees3/1
  [Perr] -> Radians to Degrees2/1
  Radians to Degrees3/1 -> P_V_comp/4  "Vel_err"
  Radians to Degrees2/1 -> P_V_comp/2  "Pos_err"
  Radians to Degrees1/1 -> P_V_comp/3  "Vel"
  Radians to Degrees4/1 -> P_V_comp/1  "Pos"
  [TQ] -> P_V_comp/5  "VTQ"
  [T] -> P_V_comp/6  "T_tot"
  PID Controller1/1 -> Sum1/2, [TQ]
